simulink model "untitled"  (R2021b)
settings: Solver=FixedStepAuto  StartTime=0  StopTime=20  FixedStep=0.001  RelTol=1e-3
model workspace (MAT data in the model file):
  v = 1
settings Model: Creator=zhu52520  LastModifiedBy=zhu52520
settings DataIOCC: ExternalInput=[t,u]

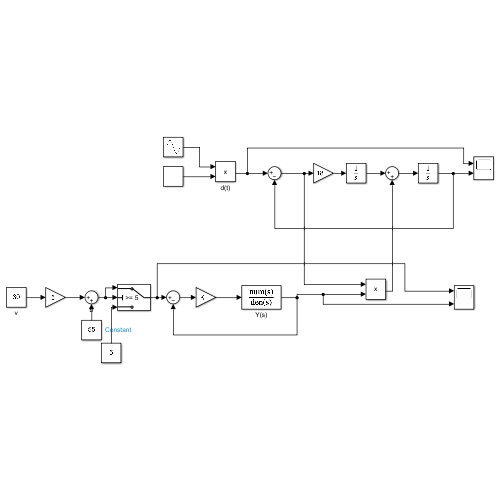
[thumbnail: Simulink's stored preview of the top-level diagram]
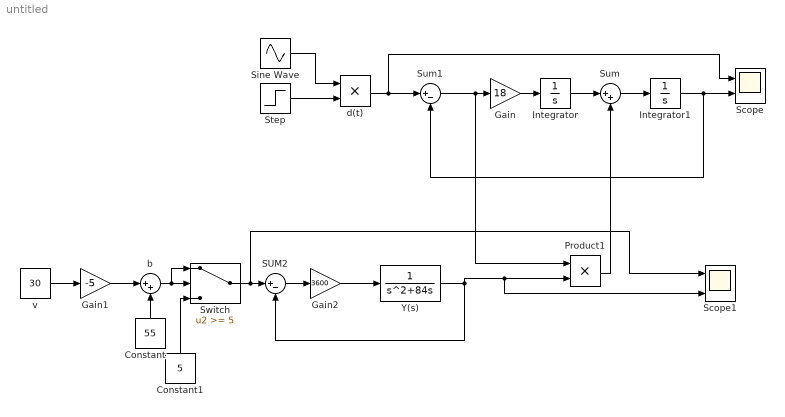
== system untitled ==
  Constant : Constant  Value=55
  Constant1 : Constant  Value=5
  Gain : Gain  Gain=18
  Gain1 : Gain  Gain=-5
  Gain2 : Gain  Gain=3600
  Integrator : Integrator  UpperSaturationLimit=10000  LowerSaturationLimit=-10000
  Integrator1 : Integrator  UpperSaturationLimit=10000  LowerSaturationLimit=-10000
  Product1 : Product
  SUM2 : Sum  Inputs=|+-
  Scope : Scope  NumInputPorts=2
  Scope1 : Scope  NumInputPorts=2
  Sine Wave : Sin  Amplitude=10  Frequency=30  SampleTime=0
  Step : Step  Time=5  Before=1  After=0  SampleTime=0
  Sum : Sum  Inputs=|++
  Sum1 : Sum  Inputs=|+-
  Switch : Switch  Threshold=5
  Y(s) : TransferFcn  Denominator=[1 84 0]
  b : Sum  Inputs=|++  OutMin=5  OutMax=200
  d(t) : Product
  v : Constant  Value=30
  wires:
  Integrator/1 -> Sum/1
  Product1/1 -> Sum/2
  Sum/1 -> Integrator1/1
  Sum1/1 -> Product1/1, Gain/1
  Integrator1/1 -> Sum1/2, Scope/2
  Step/1 -> d(t)/2
  Sine Wave/1 -> d(t)/1
  Gain/1 -> Integrator/1
  Constant/1 -> b/2
  Gain1/1 -> b/1
  d(t)/1 -> Scope/1, Sum1/1
  v/1 -> Gain1/1
  Gain2/1 -> Y(s)/1
  Y(s)/1 -> Scope1/2, Product1/2, SUM2/2
  SUM2/1 -> Gain2/1
  b/1 -> Switch/1, Switch/2
  Constant1/1 -> Switch/3
  Switch/1 -> Scope1/1, SUM2/1
